simulink model "one"  (R2020b)
settings: Solver=VariableStepAuto  StartTime=0.0  StopTime=10.0  RelTol=1e-3
settings Model: Creator=USER  LastModifiedBy=USER

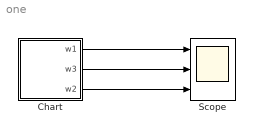
== system one ==
  Chart : Stateflow chart  TreatAsAtomicUnit=on
  Scope : Scope  NumInputPorts=3
  wires:
  Chart/1(w1) -> Scope/1
  Chart/2(w3) -> Scope/2
  Chart/3(w2) -> Scope/3

== stateflow chart one/Chart ==
  state State1
    entry:
    w3=0;
    w2=0;
    w1=0;
  state State5
    entry:
    w3=1;
    w2=0;
    w1=0;
  state State2
    entry:
    w3=0;
    w2=0;
    w1=1;
  state State3
    entry:
    w3=0;
    w2=1;
    w1=0;
  state State4
    entry:
    w3=0;
    w2=1;
    w1=1;
  (default) -> State1
  State5 -> State1 : {w1==1&&w2==0&&w3==0}
  State1 -> State2 : {w1==0&&w2==0&&w3==0}
  State4 -> State5 : {w1==0&&w2==1&&w3==1}
  State2 -> State3 : {w1==0&&w2==0&&w3==1}
  State3 -> State4 : {w1==0&&w2==1&&w3==0}
  data: w1 output; w3 output; w2 output
